simulink model "SimulacionControl"  (R2018a)
settings: Solver=VariableStepAuto  StartTime=0.0  StopTime=5  FixedStep=0.001  RelTol=1e-3
values from neighbouring files (symbols this model uses):
  Ts_control = 0.001    [A_SimulacionAnalisis.m]
undefined symbols (not defined in the file or in its folder): mcd, mci
settings Model: Creator=Richa  LastModifiedBy=richard
settings DataIOCC: ReturnWorkspaceOutputsName=tpa64da4d0_65d4_4f68_a7aa_c48a3dcc3ace
settings CodeAppCC: StateflowObjectComments=on

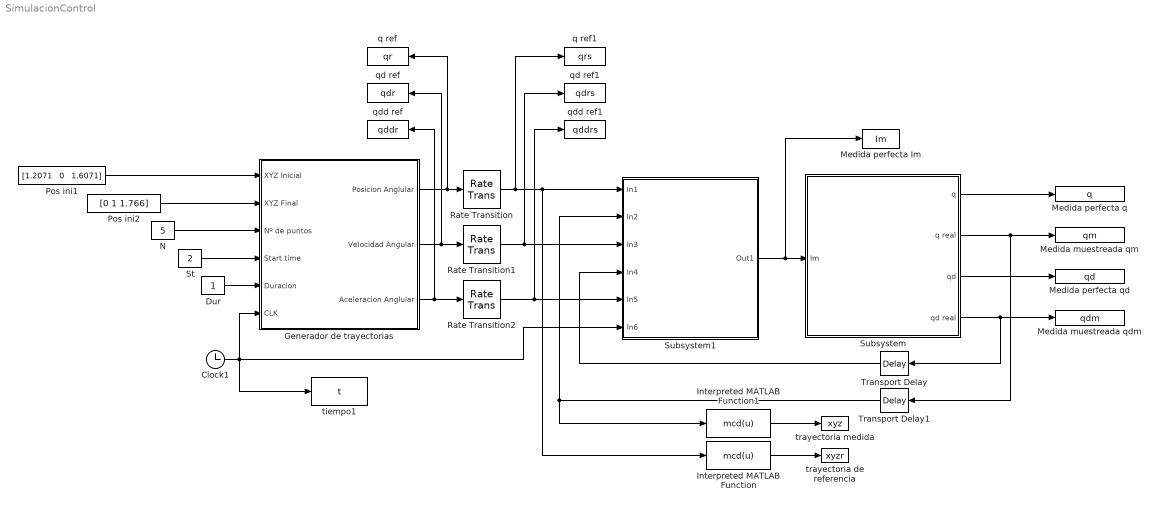
== system SimulacionControl ==
  Clock1 : Clock
  Dur : Constant
  Generador de trayectorias : Subsystem
      mask Display: image('screenshot.png');
  Interpreted MATLAB Function : MATLABFcn  MATLABFcn=mcd(u)
  Interpreted MATLAB Function1 : MATLABFcn  MATLABFcn=mcd(u)
  Medida muestreada qdm : ToWorkspace  VariableName=qdm  SampleTime=Ts_control
  Medida muestreada qm : ToWorkspace  VariableName=qm  SampleTime=Ts_control
  Medida perfecta Im : ToWorkspace  VariableName=Im
  Medida perfecta q : ToWorkspace  VariableName=q  SampleTime=-1
  Medida perfecta qd : ToWorkspace  VariableName=qd  SampleTime=-1
  N : Constant  Value=5
  Pos ini1 : Constant  Value="[1.2071   0   1.6071]"
  Pos ini2 : Constant  Value=[0 1 1.766]
  Rate Transition : RateTransition  OutPortSampleTimeMultiple=ZOH  OutPortSampleTime=Ts_reference
  Rate Transition1 : RateTransition  OutPortSampleTime=Ts_reference
  Rate Transition2 : RateTransition  OutPortSampleTime=Ts_reference
  St : Constant  Value=2
  Subsystem : Subsystem
  Subsystem1 : Subsystem  TreatAsAtomicUnit=on  SystemSampleTime=Ts_control
  Transport Delay : TransportDelay  DelayTime=1e-18
  Transport Delay1 : TransportDelay  DelayTime=1e-18  InitialOutput="mci([1.2071   0   1.6071],1)"
  q ref : ToWorkspace  VariableName=qr  SampleTime=-1
  q ref1 : ToWorkspace  VariableName=qrs
  qd ref : ToWorkspace  VariableName=qdr  SampleTime=-1
  qd ref1 : ToWorkspace  VariableName=qdrs
  qdd ref : ToWorkspace  VariableName=qddr  SampleTime=-1
  qdd ref1 : ToWorkspace  VariableName=qddrs
  tiempo1 : ToWorkspace  VariableName=t
  trayectoria de referencia : ToWorkspace  VariableName=xyzr
  trayectoria medida : ToWorkspace  VariableName=xyz
  wires:
  Pos ini2/1 -> Generador de trayectorias/2(XYZ Final)
  Pos ini1/1 -> Generador de trayectorias/1(XYZ Inicial)
  St/1 -> Generador de trayectorias/4(Start time)
  N/1 -> Generador de trayectorias/3(Nº de puntos)
  Dur/1 -> Generador de trayectorias/5(Duracion)
  Generador de trayectorias/1(" Posicion Anglular") -> Rate Transition/1, q ref/1
  Generador de trayectorias/2(Velocidad Angular) -> Rate Transition1/1, qd ref/1
  Generador de trayectorias/3(Aceleracion Anglular) -> Rate Transition2/1, qdd ref/1
  Interpreted MATLAB Function/1 -> trayectoria de referencia/1
  Rate Transition/1 -> Interpreted MATLAB Function/1, Subsystem1/1(In1), q ref1/1
  Interpreted MATLAB Function1/1 -> trayectoria medida/1
  Subsystem/3(qd) -> Medida perfecta qd/1
  Subsystem/1(q) -> Medida perfecta q/1
  Subsystem/4(qd real) -> Transport Delay/1, Medida muestreada qdm/1
  Rate Transition2/1 -> Subsystem1/5(In5), qdd ref1/1
  Clock1/1 -> Subsystem1/6(In6), tiempo1/1, Generador de trayectorias/6(CLK)
  Subsystem/2(q real) -> Transport Delay1/1, Medida muestreada qm/1
  Rate Transition1/1 -> Subsystem1/3(In3), qd ref1/1
  Subsystem1/1(Out1) -> Subsystem/1(Im), Medida perfecta Im/1
  Transport Delay1/1 -> Interpreted MATLAB Function1/1, Subsystem1/2(In2)
  Transport Delay/1 -> Subsystem1/4(In4)

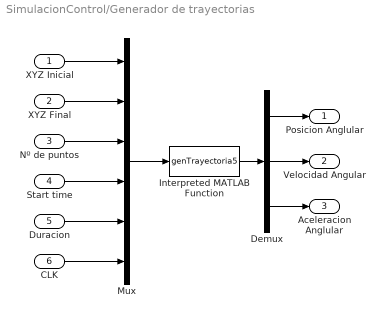
== system SimulacionControl/Generador de trayectorias ==
  XYZ Inicial : Inport
  XYZ Final : Inport  Port=2
  Nº de puntos : Inport  Port=3
  Start time : Inport  Port=4
  Duracion : Inport  Port=5
  CLK : Inport  Port=6
  Demux : Demux  Outputs=3
  Interpreted MATLAB Function : MATLABFcn  MATLABFcn=genTrayectoria5  OutputDimensions=9
  Mux : Mux  Inputs=6
  " Posicion Anglular" : Outport  PortDimensions=3
  Velocidad Angular : Outport  Port=2  PortDimensions=3
  Aceleracion Anglular : Outport  Port=3  PortDimensions=3
  wires:
  Demux/3 -> Aceleracion Anglular/1
  Mux/1 -> Interpreted MATLAB Function/1
  Nº de puntos/1 -> Mux/3
  CLK/1 -> Mux/6
  Start time/1 -> Mux/4
  Interpreted MATLAB Function/1 -> Demux/1
  Duracion/1 -> Mux/5
  XYZ Final/1 -> Mux/2
  XYZ Inicial/1 -> Mux/1
  Demux/1 -> " Posicion Anglular"/1
  Demux/2 -> Velocidad Angular/1

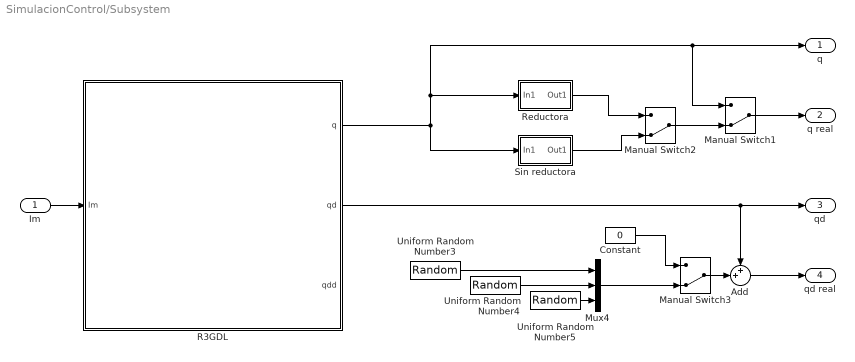
== system SimulacionControl/Subsystem ==
  Im : Inport
  Add : Sum  Inputs=++|
  Constant : Constant  Value=0
  Manual Switch1 : ManualSwitch  CurrentSetting=0
  Manual Switch2 : ManualSwitch  CurrentSetting=0
  Manual Switch3 : ManualSwitch  CurrentSetting=0
  Mux4 : Mux  Inputs=3
  R3GDL : Subsystem  mask(Control y Programación de Robots (4 GIERM)){NGrupo=15, q1_ini=[1 0 0]*mci([1.2071   0   1.6071],1), q2_ini=[0 1 0]*mci([1.2071   0   1.6071],0), q3_ini=[0 0 1]*mci([1.2071   0   1.6071],0), Bl_q1=off, Bl_q2=off, Bl_q3=off, AccionamientoDirecto=on}
      mask prompts: NGrupo "Nº de GRUPO"; q1_ini "q1 inicial  (rad)"; q2_ini "q2 inicial (rad)"; q3_ini "q3_inicial (rad)"; Bl_q1 "Bloqueo q1"; Bl_q2 "Bloqueo q2"; Bl_q3 "Bloqueo q3"; AccionamientoDirecto "Accionamiento directo"
      mask help: Robot de 3 grados de libertad RRR
      mask Display:
      | image(imread('R3GDL_RRR.JPG'));
      | port_label('output', 1, 'q');
      | port_label('output', 2, 'qd');
      | port_label('output', 3, 'qdd');
      | port_label('input', 1, 'Im')
  Reductora : Subsystem
  Sin reductora : Subsystem
  Uniform Random Number3 : UniformRandomNumber  Minimum=-(1500*2*pi/60)*(0.01/50)  Maximum=(1500*2*pi/60)*(0.01/50)  SampleTime=0.001
  Uniform Random Number4 : UniformRandomNumber  Minimum=-(1500*2*pi/60)*(0.01/30)  Maximum=(1500*2*pi/60)*(0.01/30)  SampleTime=0.001
  Uniform Random Number5 : UniformRandomNumber  Minimum=-(1500*2*pi/60)*(0.01/15)  Maximum=(1500*2*pi/60)*(0.01/15)  SampleTime=0.001
  q : Outport
  q real : Outport  Port=2
  qd : Outport  Port=3
  qd real : Outport  Port=4
  wires:
  Im/1 -> R3GDL/1(Im)
  R3GDL/2(qd) -> Add/1, qd/1
  Add/1 -> qd real/1
  R3GDL/1(q) -> Manual Switch1/1, q/1, Reductora/1(In1), Sin reductora/1(In1)
  Manual Switch1/1 -> q real/1
  Uniform Random Number3/1 -> Mux4/1
  Uniform Random Number4/1 -> Mux4/2
  Uniform Random Number5/1 -> Mux4/3
  Mux4/1 -> Manual Switch3/2
  Manual Switch3/1 -> Add/2
  Constant/1 -> Manual Switch3/1
  Reductora/1(Out1) -> Manual Switch2/1
  Sin reductora/1(Out1) -> Manual Switch2/2
  Manual Switch2/1 -> Manual Switch1/2

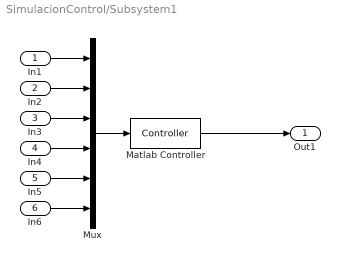
== system SimulacionControl/Subsystem1 ==
  In1 : Inport
  In2 : Inport  Port=2
  In3 : Inport  Port=3
  In4 : Inport  Port=4
  In5 : Inport  Port=5
  In6 : Inport  Port=6
  "Matlab Controller " : MATLABFcn  MATLABFcn=Controller
  Mux : Mux  Inputs=6
  Out1 : Outport
  wires:
  In1/1 -> Mux/1
  "Matlab Controller "/1 -> Out1/1
  Mux/1 -> "Matlab Controller "/1
  In2/1 -> Mux/2
  In3/1 -> Mux/3
  In4/1 -> Mux/4
  In5/1 -> Mux/5
  In6/1 -> Mux/6

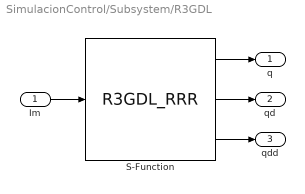
== system SimulacionControl/Subsystem/R3GDL ==
  Im : Inport
  S-Function : S-Function  FunctionName=R3GDL_RRR  Parameters=[q1_ini; q2_ini; q3_ini]; [Bl_q1; Bl_q2; Bl_q3]; AccionamientoDirecto; NGrupo  SFunctionDeploymentMode=off  EnableBusSupport=off
  q : Outport
  qd : Outport  Port=2
  qdd : Outport  Port=3
  wires:
  Im/1 -> S-Function/1
  S-Function/1 -> q/1
  S-Function/2 -> qd/1
  S-Function/3 -> qdd/1

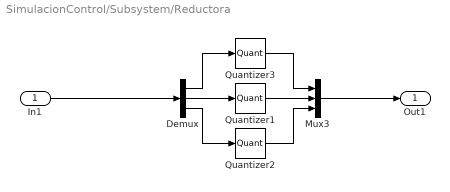
== system SimulacionControl/Subsystem/Reductora ==
  In1 : Inport
  Demux : Demux  Outputs=3
  Mux3 : Mux  Inputs=3
  Quantizer1 : Quantizer  QuantizationInterval=2*pi/1024/30
  Quantizer2 : Quantizer  QuantizationInterval=2*pi/1024/15
  Quantizer3 : Quantizer  QuantizationInterval=2*pi/1024/50
  Out1 : Outport
  wires:
  Demux/1 -> Quantizer3/1
  In1/1 -> Demux/1
  Quantizer1/1 -> Mux3/2
  Quantizer3/1 -> Mux3/1
  Demux/2 -> Quantizer1/1
  Quantizer2/1 -> Mux3/3
  Mux3/1 -> Out1/1
  Demux/3 -> Quantizer2/1

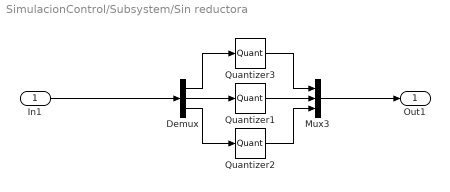
== system SimulacionControl/Subsystem/Sin reductora ==
  In1 : Inport
  Demux : Demux  Outputs=3
  Mux3 : Mux  Inputs=3
  Quantizer1 : Quantizer  QuantizationInterval=2*pi/1024
  Quantizer2 : Quantizer  QuantizationInterval=2*pi/1024
  Quantizer3 : Quantizer  QuantizationInterval=2*pi/1024
  Out1 : Outport
  wires:
  Demux/3 -> Quantizer2/1
  Mux3/1 -> Out1/1
  Quantizer2/1 -> Mux3/3
  Demux/2 -> Quantizer1/1
  Quantizer3/1 -> Mux3/1
  Quantizer1/1 -> Mux3/2
  In1/1 -> Demux/1
  Demux/1 -> Quantizer3/1
